simulink model "two_equation"  (R2019a)
settings: Solver=VariableStepAuto  StartTime=0.0  StopTime=500  RelTol=1e-3
libraries: simulink x2
settings Model: Creator=Mohamed Nofal  LastModifiedBy=Mohamed Nofal

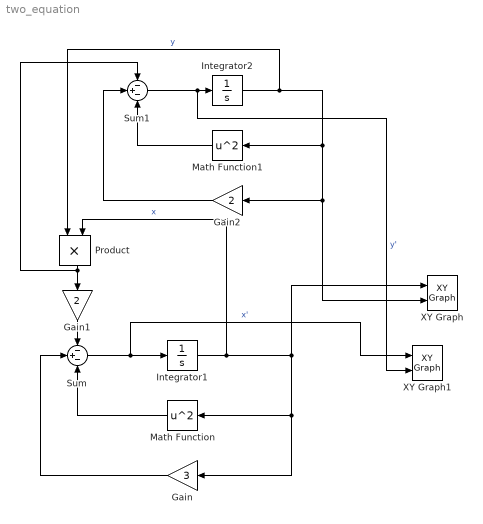
== system two_equation ==
  Gain : Gain  Gain=3
  Gain1 : Gain  Gain=2
  Gain2 : Gain  Gain=2
  Integrator1 : Integrator  InitialCondition=0.5
  Integrator2 : Integrator  InitialCondition=0.5
  Math Function : Math  Operator=square  SaturateOnIntegerOverflow=on
  Math Function1 : Math  Operator=square  SaturateOnIntegerOverflow=on
  Product : Product
  Sum : Sum  Inputs=-+-
  Sum1 : Sum  Inputs=-+-
  XY Graph : simulink/Sinks/XY Graph  xmin=-10  xmax=10  ymin=-10  ymax=10  st=-1
  XY Graph1 : simulink/Sinks/XY Graph  xmin=-1  xmax=1  ymin=-1  ymax=1  st=-1
  wires:
  Integrator1/1 -> Product/2, XY Graph/1, Math Function/1, Gain/1  "x"
  Sum/1 -> XY Graph1/1, Integrator1/1  "x'"
  Gain/1 -> Sum/2
  Math Function/1 -> Sum/3
  Gain1/1 -> Sum/1
  Sum1/1 -> XY Graph1/2, Integrator2/1  "y'"
  Integrator2/1 -> Product/1, XY Graph/2, Gain2/1, Math Function1/1  "y"
  Gain2/1 -> Sum1/2
  Math Function1/1 -> Sum1/3
  Product/1 -> Sum1/1, Gain1/1
